simulink model "antiWindup2"  (R2019a)
settings: Solver=VariableStepAuto  StartTime=0.0  StopTime=30  RelTol=1e-3
values from neighbouring files (symbols this model uses):
  Ki = 2    [mainAntiWindup1.m]    (also in mainAntiWindup2.m; mainBumpless.m; mainLimAzioneDerivativa.m = 1; mainWindupIntegrale.m)
  Kp = 2    [mainAntiWindup1.m]    (also in mainAntiWindup2.m; mainBumpless.m; mainLimAzioneDerivativa.m; mainWindupIntegrale.m = 0)
  UM = 1.05    [mainAntiWindup1.m]    (also in mainAntiWindup2.m; mainBumpless.m = inf; mainWindupIntegrale.m)
settings Model: Creator=adria  LastModifiedBy=adria

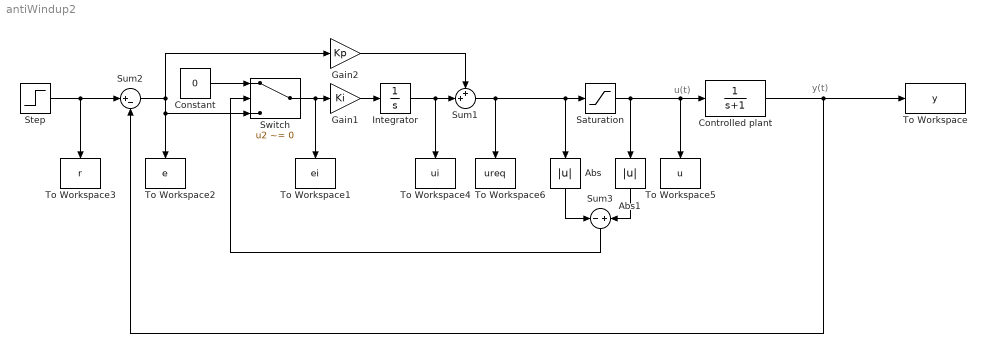
== system antiWindup2 ==
  note: u(t)
  note: y(t)
  Abs : Abs
  Abs1 : Abs
  Constant : Constant  Value=0
  Controlled plant : TransferFcn  Denominator=[1 1]
  Gain1 : Gain  Gain=Ki
  Gain2 : Gain  Gain=Kp
  Integrator : Integrator
  Saturation : Saturate  UpperLimit=UM  LowerLimit=-UM
  Step : Step  SampleTime=0
  Sum1 : Sum  Inputs=++|
  Sum2 : Sum  Inputs=|+-
  Sum3 : Sum  Inputs=-+
  Switch : Switch  Criteria=u2 ~= 0
  To Workspace : ToWorkspace  VariableName=y  SaveFormat=Structure With Time  SampleTime=-1
  To Workspace1 : ToWorkspace  VariableName=ei  SaveFormat=Structure With Time  SampleTime=-1
  To Workspace2 : ToWorkspace  VariableName=e  SaveFormat=Structure With Time  SampleTime=-1
  To Workspace3 : ToWorkspace  VariableName=r  SaveFormat=Structure With Time  SampleTime=-1
  To Workspace4 : ToWorkspace  VariableName=ui  SaveFormat=Structure With Time  SampleTime=-1
  To Workspace5 : ToWorkspace  VariableName=u  SaveFormat=Structure With Time  SampleTime=-1
  To Workspace6 : ToWorkspace  VariableName=ureq  SaveFormat=Structure With Time  SampleTime=-1
  wires:
  Step/1 -> To Workspace3/1, Sum2/1
  Integrator/1 -> Sum1/2, To Workspace4/1
  Gain1/1 -> Integrator/1
  Controlled plant/1 -> Sum2/2, To Workspace/1
  Sum2/1 -> Switch/3, To Workspace2/1, Gain2/1
  Saturation/1 -> Abs1/1, To Workspace5/1, Controlled plant/1
  Sum1/1 -> To Workspace6/1, Abs/1, Saturation/1
  Gain2/1 -> Sum1/1
  Switch/1 -> To Workspace1/1, Gain1/1
  Abs1/1 -> Sum3/2
  Abs/1 -> Sum3/1
  Sum3/1 -> Switch/2
  Constant/1 -> Switch/1
